simulink model "Simulink_work"  (R2022b)
settings: Solver=VariableStepAuto  StartTime=0.0  StopTime=10  RelTol=1e-3
values from neighbouring files (symbols this model uses):
  A = [0 1 ... (first row only)    [Matlab_.m]    (also in THISISTHEMAINMATLABFIEL.m = A_new)
  B = [0; 239.4]    [Matlab_.m]    (also in THISISTHEMAINMATLABFIEL.m = [B; 0])
  C = [0 1]    [Matlab_.m]    (also in THISISTHEMAINMATLABFIEL.m = [0 0.1 0])
  K = place(A, B, desired_poles)    [Matlab_.m]    (also in THISISTHEMAINMATLABFIEL.m = K_IntegralControl(1:2))
  K1 = K(1)    [Matlab_.m]
  KK = [0 K(2)]    [Matlab_.m]
settings Model: SimulationMode=accelerator  Creator=havso  LastModifiedBy=havso

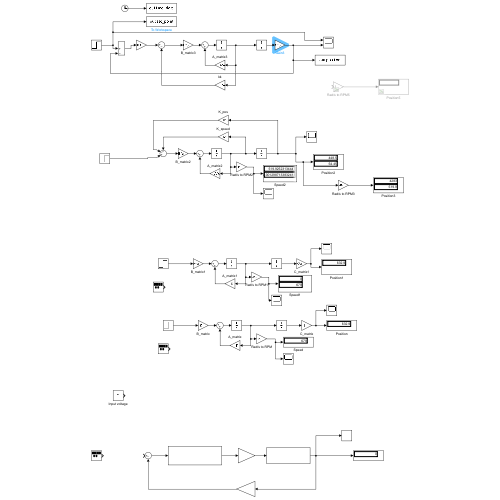
[thumbnail: Simulink's stored preview of the top-level diagram]
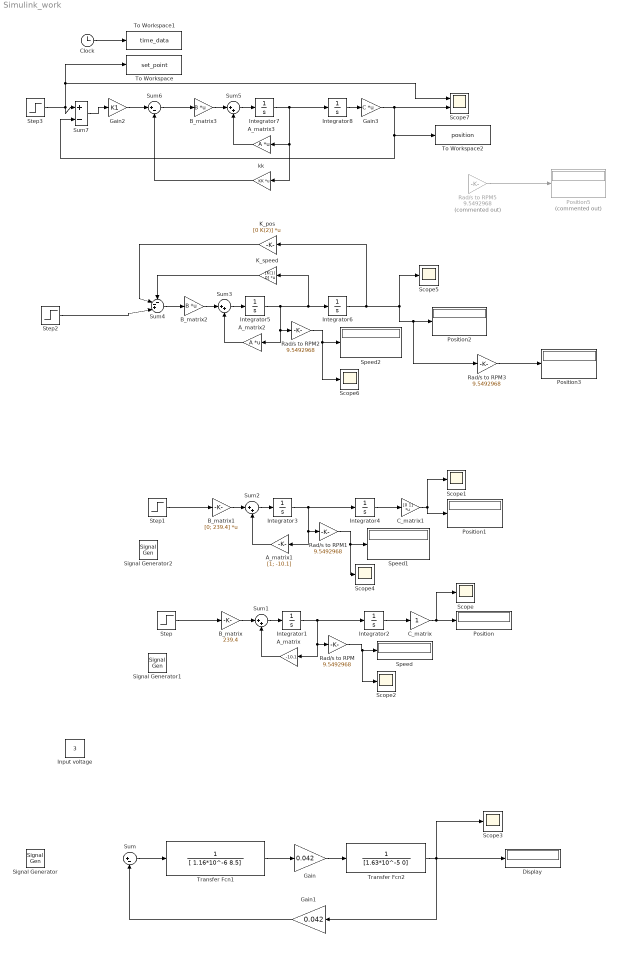
== system Simulink_work ==
  A_matrix : Gain  Gain=-10.1
  A_matrix1 : Gain  Gain=[1; -10.1]
  A_matrix2 : Gain  Gain=A  Multiplication=Matrix(K*u)
  A_matrix3 : Gain  Gain=A  Multiplication=Matrix(K*u)
  B_matrix : Gain  Gain=239.4
  B_matrix1 : Gain  Gain=[0; 239.4]  Multiplication=Matrix(K*u)
  B_matrix2 : Gain  Gain=B  Multiplication=Matrix(K*u)
  B_matrix3 : Gain  Gain=B  Multiplication=Matrix(K*u)
  C_matrix : Gain
  C_matrix1 : Gain  Gain=[0 1]  Multiplication=Matrix(K*u)
  Clock : Clock
  Display : Display
  Gain : Gain  Gain=0.042
  Gain1 : Gain  Gain=0.042
  Gain2 : Gain  Gain=K1
  Gain3 : Gain  Gain=C  Multiplication=Matrix(K*u)
  Input voltage : Constant  Value=3
  Integrator{1..8} (8 alike) : Integrator
  K_pos : Gain  Gain=[0 K(2)]  Multiplication=Matrix(K*u)
  K_speed : Gain  Gain=[K(1) 0]  Multiplication=Matrix(K*u)
  Position{,1..3} (4 alike) : Display
  Position5 : Display  Commented=on
  Rad/s to RPM{,1..3} (4 alike) : Gain  Gain=9.5492968
  Rad/s to RPM5 : Gain  Commented=on  Gain=9.5492968
  Scope{,1..6} (7 alike) : Scope
  Scope7 : Scope  NumInputPorts=2
  Signal Generator : SignalGenerator  Amplitude=3  Units=rad/sec
  Signal Generator1 : SignalGenerator  Amplitude=3  Units=rad/sec
  Signal Generator2 : SignalGenerator  Amplitude=3  Units=rad/sec
  Speed : Display
  Speed1 : Display
  Speed2 : Display
  Step{,1..3} (4 alike) : Step  After=3  SampleTime=0
  Sum : Sum  Inputs=|+-
  Sum{1..3,5} (4 alike) : Sum  Inputs=|++
  Sum4 : Sum  Inputs=--+|
  Sum6 : Sum  Inputs=|+-
  Sum7 : Sum  Inputs=|+-
  To Workspace : ToWorkspace  VariableName=set_point  SampleTime=-1
  To Workspace1 : ToWorkspace  VariableName=time_data  SampleTime=-1
  To Workspace2 : ToWorkspace  VariableName=position  SampleTime=-1
  Transfer Fcn1 : TransferFcn  Denominator=[ 1.16*10^-6 8.5]
  Transfer Fcn2 : TransferFcn  Denominator=[1.63*10^-5 0]
  kk : Gain  Gain=KK  Multiplication=Matrix(K*u)
  wires:
  Sum/1 -> Transfer Fcn1/1
  Transfer Fcn1/1 -> Gain/1
  Gain/1 -> Transfer Fcn2/1
  Transfer Fcn2/1 -> Scope3/1, Gain1/1, Display/1
  Gain1/1 -> Sum/2
  Sum1/1 -> Integrator1/1
  B_matrix/1 -> Sum1/1
  A_matrix/1 -> Sum1/2
  Integrator2/1 -> C_matrix/1
  Integrator1/1 -> Rad/s to RPM/1, A_matrix/1, Integrator2/1
  C_matrix/1 -> Scope/1, Position/1
  Rad/s to RPM/1 -> Scope2/1, Speed/1
  Step/1 -> B_matrix/1
  Integrator4/1 -> C_matrix1/1
  C_matrix1/1 -> Scope1/1, Position1/1
  Rad/s to RPM1/1 -> Scope4/1, Speed1/1
  Step1/1 -> B_matrix1/1
  Integrator3/1 -> Rad/s to RPM1/1, A_matrix1/1, Integrator4/1
  B_matrix1/1 -> Sum2/1
  Sum2/1 -> Integrator3/1
  A_matrix1/1 -> Sum2/2
  Integrator6/1 -> K_pos/1, Scope5/1, Rad/s to RPM3/1, Position2/1
  Sum3/1 -> Integrator5/1
  A_matrix2/1 -> Sum3/2
  B_matrix2/1 -> Sum3/1
  Integrator5/1 -> Rad/s to RPM2/1, A_matrix2/1, K_speed/1, Integrator6/1
  Rad/s to RPM2/1 -> Scope6/1, Speed2/1
  K_speed/1 -> Sum4/1
  Sum4/1 -> B_matrix2/1
  Step2/1 -> Sum4/3
  K_pos/1 -> Sum4/2
  Rad/s to RPM3/1 -> Position3/1
  Sum6/1 -> B_matrix3/1
  Integrator7/1 -> kk/1, A_matrix3/1, Integrator8/1
  Sum5/1 -> Integrator7/1
  B_matrix3/1 -> Sum5/1
  A_matrix3/1 -> Sum5/2
  Rad/s to RPM5/1 -> Position5/1
  kk/1 -> Sum6/2
  Sum7/1 -> Gain2/1
  Step3/1 -> To Workspace/1, Scope7/1, Sum7/1
  Gain2/1 -> Sum6/1
  Integrator8/1 -> Gain3/1
  Gain3/1 -> To Workspace2/1, Sum7/2, Scope7/2
  Clock/1 -> To Workspace1/1
